simulink model "BehKettleBehavior"  (R2026a)
settings: Solver=VariableStepAuto
settings Model: DataDictionary=PhysicalInterfaces.sldd  Creator=sarah  LastModifiedBy=sarah

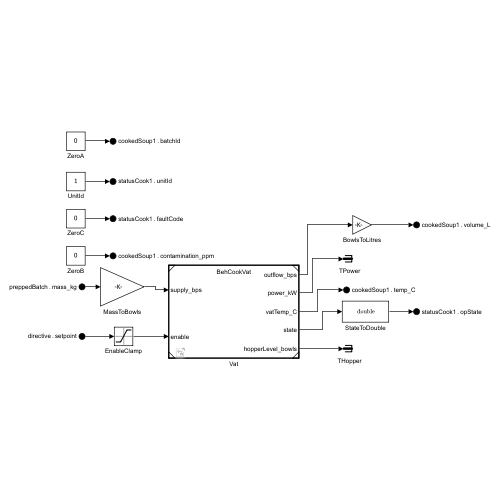
[thumbnail: Simulink's stored preview of the top-level diagram]
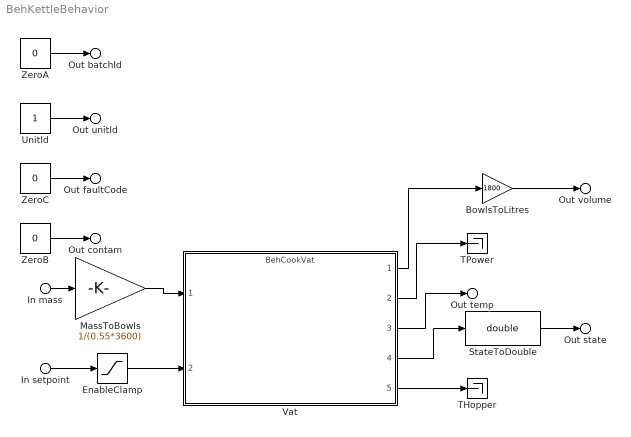
== system BehKettleBehavior ==
  In mass : Inport  PortName=preppedBatch  Element=mass_kg
  In setpoint : Inport  Port=2  PortName=directive  Element=setpoint
  BowlsToLitres : Gain  Gain=1800
  EnableClamp : Saturate  UpperLimit=1  LowerLimit=0
  MassToBowls : Gain  Gain=1/(0.55*3600)
  StateToDouble : DataTypeConversion  OutDataTypeStr=double  SaturateOnIntegerOverflow=off  RndMeth=Floor
  THopper : Terminator
  TPower : Terminator
  UnitId : Constant
  Vat : ModelReference  ModelNameDialog=BehCookVat  UsingDefaultArgumentValue=0,0,0,0,0,0,0,0  SimulationMode=Normal  ModelReferenceVersion=1.7
  ZeroA : Constant  Value=0
  ZeroB : Constant  Value=0
  ZeroC : Constant  Value=0
  Out batchId : Outport  PortName=cookedSoup1  Element=batchId
  Out volume : Outport  PortName=cookedSoup1  Element=volume_L
  Out temp : Outport  PortName=cookedSoup1  Element=temp_C
  Out contam : Outport  PortName=cookedSoup1  Element=contamination_ppm
  Out unitId : Outport  Port=2  PortName=statusCook1  Element=unitId
  Out state : Outport  Port=2  PortName=statusCook1  Element=opState
  Out faultCode : Outport  Port=2  PortName=statusCook1  Element=faultCode
  wires:
  ZeroC/1 -> Out faultCode/1
  Vat/4 -> StateToDouble/1
  Vat/3 -> Out temp/1
  ZeroA/1 -> Out batchId/1
  UnitId/1 -> Out unitId/1
  Vat/5 -> THopper/1
  ZeroB/1 -> Out contam/1
  In mass/1 -> MassToBowls/1
  MassToBowls/1 -> Vat/1
  In setpoint/1 -> EnableClamp/1
  EnableClamp/1 -> Vat/2
  Vat/1 -> BowlsToLitres/1
  Vat/2 -> TPower/1
  BowlsToLitres/1 -> Out volume/1
  StateToDouble/1 -> Out state/1
